simulink model "odev2"  (R2014a)
settings: Solver=ode45  StartTime=0.0  StopTime=10.0  RelTol=1e-3
undefined symbols (not defined in the file): gray, Rec, SDTV
libraries: visionconversions x18, visionsinks x14, visionsources x1
settings Model: Creator=bizimakin  LastModifiedBy=bizimakin
settings DebuggingCC: UnderspecifiedInitializationDetection=Classic  StateNameClashWarn=warning

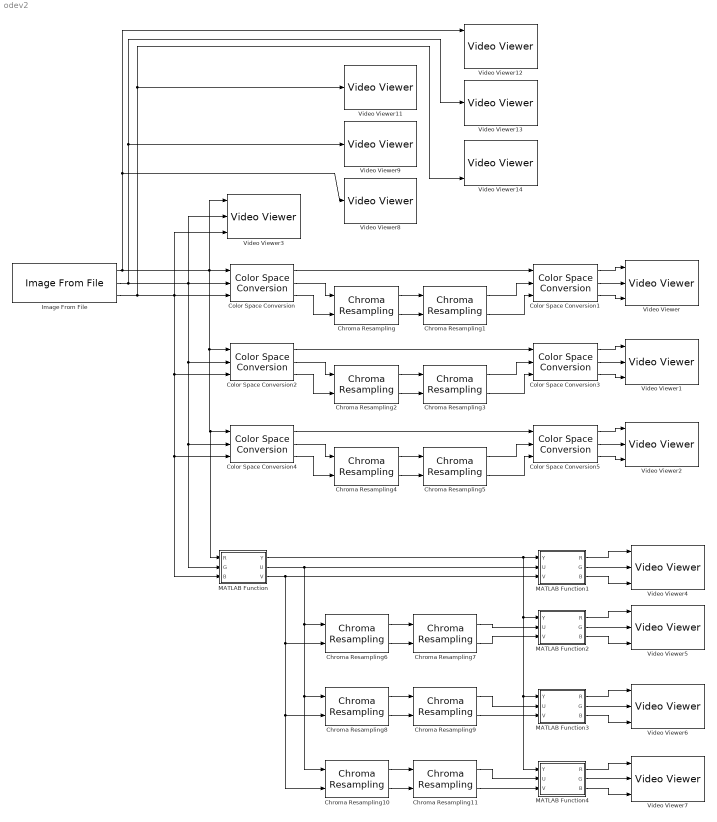
== system odev2 ==
  Chroma Resampling : visionconversions/Chroma Resampling  resampling=4:4:4 to 4:2:2  interpolation=pixel replication  antialiasing=Default  hcoeff=[0.2 0.6 0.2]  vcoeff=[0.5 0.5]  isInputTransposed=off
  Chroma Resampling1 : visionconversions/Chroma Resampling  resampling=4:2:2 to 4:4:4  interpolation=linear  antialiasing=Default  hcoeff=[0.2 0.6 0.2]  vcoeff=[0.5 0.5]  isInputTransposed=off
  Chroma Resampling10 : visionconversions/Chroma Resampling  resampling=4:4:4 to 4:2:0 (MPEG1)  interpolation=pixel replication  antialiasing=Default  hcoeff=[0.2 0.6 0.2]  vcoeff=[0.5 0.5]  isInputTransposed=off
  Chroma Resampling11 : visionconversions/Chroma Resampling  resampling=4:2:0 (MPEG1) to 4:4:4  interpolation=linear  antialiasing=Default  hcoeff=[0.2 0.6 0.2]  vcoeff=[0.5 0.5]  isInputTransposed=off
  Chroma Resampling2 : visionconversions/Chroma Resampling  resampling=4:4:4 to 4:1:1  interpolation=pixel replication  antialiasing=Default  hcoeff=[0.2 0.6 0.2]  vcoeff=[0.5 0.5]  isInputTransposed=off
  Chroma Resampling3 : visionconversions/Chroma Resampling  resampling=4:1:1 to 4:4:4  interpolation=linear  antialiasing=Default  hcoeff=[0.2 0.6 0.2]  vcoeff=[0.5 0.5]  isInputTransposed=off
  Chroma Resampling4 : visionconversions/Chroma Resampling  resampling=4:4:4 to 4:2:0 (MPEG1)  interpolation=pixel replication  antialiasing=Default  hcoeff=[0.2 0.6 0.2]  vcoeff=[0.5 0.5]  isInputTransposed=off
  Chroma Resampling5 : visionconversions/Chroma Resampling  resampling=4:2:0 (MPEG1) to 4:4:4  interpolation=linear  antialiasing=Default  hcoeff=[0.2 0.6 0.2]  vcoeff=[0.5 0.5]  isInputTransposed=off
  Chroma Resampling6 : visionconversions/Chroma Resampling  resampling=4:4:4 to 4:2:2  interpolation=pixel replication  antialiasing=Default  hcoeff=[0.2 0.6 0.2]  vcoeff=[0.5 0.5]  isInputTransposed=off
  Chroma Resampling7 : visionconversions/Chroma Resampling  resampling=4:2:2 to 4:4:4  interpolation=linear  antialiasing=Default  hcoeff=[0.2 0.6 0.2]  vcoeff=[0.5 0.5]  isInputTransposed=off
  Chroma Resampling8 : visionconversions/Chroma Resampling  resampling=4:4:4 to 4:1:1  interpolation=pixel replication  antialiasing=Default  hcoeff=[0.2 0.6 0.2]  vcoeff=[0.5 0.5]  isInputTransposed=off
  Chroma Resampling9 : visionconversions/Chroma Resampling  resampling=4:1:1 to 4:4:4  interpolation=linear  antialiasing=Default  hcoeff=[0.2 0.6 0.2]  vcoeff=[0.5 0.5]  isInputTransposed=off
  Color Space Conversion : visionconversions/Color Space  Conversion  conversion=Obsolete  conversionActive=R'G'B' to Y'CbCr  wp_str=D65  rec=Rec. 601 (SDTV)  sys=1125/60/2:1  imagePorts=Separate color signals
  Color Space Conversion1 : visionconversions/Color Space  Conversion  conversion=Obsolete  conversionActive=Y'CbCr to R'G'B'  wp_str=D65  rec=Rec. 601 (SDTV)  sys=1125/60/2:1  imagePorts=Separate color signals
  Color Space Conversion2 : visionconversions/Color Space  Conversion  conversion=Obsolete  conversionActive=R'G'B' to Y'CbCr  wp_str=D65  rec=Rec. 601 (SDTV)  sys=1125/60/2:1  imagePorts=Separate color signals
  Color Space Conversion3 : visionconversions/Color Space  Conversion  conversion=Obsolete  conversionActive=Y'CbCr to R'G'B'  wp_str=D65  rec=Rec. 601 (SDTV)  sys=1125/60/2:1  imagePorts=Separate color signals
  Color Space Conversion4 : visionconversions/Color Space  Conversion  conversion=Obsolete  conversionActive=R'G'B' to Y'CbCr  wp_str=D65  rec=Rec. 601 (SDTV)  sys=1125/60/2:1  imagePorts=Separate color signals
  Color Space Conversion5 : visionconversions/Color Space  Conversion  conversion=Obsolete  conversionActive=Y'CbCr to R'G'B'  wp_str=D65  rec=Rec. 601 (SDTV)  sys=1125/60/2:1  imagePorts=Separate color signals
  Image From File : visionsources/Image From File  Tag=vipblks_nd  FileName=C:\Users\bizimakin\Desktop\parrots.jpg  imagePorts=Separate color signals  Ts=inf  ImageDataType=double  Signed=on  WordLength=16  sdImageDataType=uint(8)  FractionLengthMode=User-defined  FractionLength=15  OutPortLabels=R|G|B
  MATLAB Function : MATLAB Function  TreatAsAtomicUnit=on
  MATLAB Function1 : MATLAB Function  TreatAsAtomicUnit=on
  MATLAB Function2 : MATLAB Function  TreatAsAtomicUnit=on
  MATLAB Function3 : MATLAB Function  TreatAsAtomicUnit=on
  MATLAB Function4 : MATLAB Function  TreatAsAtomicUnit=on
  Video Viewer{,12..14} (4 alike) : visionsinks/Video Viewer  inputType=Obsolete7b  imagePorts=Separate color signals  useColorMap=off  colormapValue=gray(256)  specRange=off  minInputVal=0  maxInputVal=255  FigPos=[193 561 410 300]  AxisZoom=on  trueSizedOnce=off  OpenAtMdlStart=on  DefaultConfigurationName=vipscopes.VideoViewerScopeCfg
  Video Viewer1 : visionsinks/Video Viewer  inputType=Obsolete7b  imagePorts=Separate color signals  useColorMap=off  colormapValue=gray(256)  specRange=off  minInputVal=0  maxInputVal=255  FigPos=[390 779 410 300]  AxisZoom=on  trueSizedOnce=off  OpenAtMdlStart=on  DefaultConfigurationName=vipscopes.VideoViewerScopeCfg
  Video Viewer11 : visionsinks/Video Viewer  inputType=Obsolete7b  imagePorts=One multidimensional signal  useColorMap=off  colormapValue=gray(256)  specRange=off  minInputVal=0  maxInputVal=255  FigPos=[787 651 410 300]  AxisZoom=on  trueSizedOnce=off  OpenAtMdlStart=on  DefaultConfigurationName=vipscopes.VideoViewerScopeCfg
  Video Viewer{2,4..7} (5 alike) : visionsinks/Video Viewer  inputType=Obsolete7b  imagePorts=Separate color signals  useColorMap=off  colormapValue=gray(256)  specRange=off  minInputVal=0  maxInputVal=255  FigPos=[663 467 410 300]  AxisZoom=on  trueSizedOnce=off  OpenAtMdlStart=on  DefaultConfigurationName=vipscopes.VideoViewerScopeCfg
  Video Viewer3 : visionsinks/Video Viewer  inputType=Obsolete7b  imagePorts=Separate color signals  useColorMap=off  colormapValue=gray(256)  specRange=off  minInputVal=0  maxInputVal=255  FigPos=[787 651 410 300]  AxisZoom=on  trueSizedOnce=off  OpenAtMdlStart=on  DefaultConfigurationName=vipscopes.VideoViewerScopeCfg
  Video Viewer8 : visionsinks/Video Viewer  inputType=Obsolete7b  imagePorts=One multidimensional signal  useColorMap=off  colormapValue=gray(256)  specRange=off  minInputVal=0  maxInputVal=255  FigPos=[308 631 410 300]  AxisZoom=on  trueSizedOnce=off  OpenAtMdlStart=on  DefaultConfigurationName=vipscopes.VideoViewerScopeCfg
  Video Viewer9 : visionsinks/Video Viewer  inputType=Obsolete7b  imagePorts=One multidimensional signal  useColorMap=off  colormapValue=gray(256)  specRange=off  minInputVal=0  maxInputVal=255  FigPos=[787 651 410 300]  AxisZoom=on  trueSizedOnce=off  OpenAtMdlStart=on  DefaultConfigurationName=vipscopes.VideoViewerScopeCfg
  wires:
  Color Space Conversion/1 -> Color Space Conversion1/1
  Color Space Conversion/2 -> Chroma Resampling/1
  Color Space Conversion/3 -> Chroma Resampling/2
  Color Space Conversion1/1 -> Video Viewer/1
  Chroma Resampling/1 -> Chroma Resampling1/1
  Chroma Resampling/2 -> Chroma Resampling1/2
  Color Space Conversion1/2 -> Video Viewer/2
  Color Space Conversion1/3 -> Video Viewer/3
  Chroma Resampling1/1 -> Color Space Conversion1/2
  Chroma Resampling1/2 -> Color Space Conversion1/3
  Image From File/2 -> Video Viewer9/1, Video Viewer13/2, Video Viewer3/2, MATLAB Function/2(G), Color Space Conversion4/2, Color Space Conversion2/2, Color Space Conversion/2
  Image From File/3 -> Video Viewer14/3, Video Viewer11/1, Video Viewer3/3, MATLAB Function/3(B), Color Space Conversion4/3, Color Space Conversion2/3, Color Space Conversion/3
  Image From File/1 -> Video Viewer12/1, Video Viewer8/1, Video Viewer3/1, MATLAB Function/1(R), Color Space Conversion4/1, Color Space Conversion2/1, Color Space Conversion/1
  Color Space Conversion2/1 -> Color Space Conversion3/1
  Color Space Conversion2/2 -> Chroma Resampling2/1
  Color Space Conversion2/3 -> Chroma Resampling2/2
  Color Space Conversion3/1 -> Video Viewer1/1
  Chroma Resampling2/1 -> Chroma Resampling3/1
  Chroma Resampling2/2 -> Chroma Resampling3/2
  Color Space Conversion3/2 -> Video Viewer1/2
  Color Space Conversion3/3 -> Video Viewer1/3
  Chroma Resampling3/1 -> Color Space Conversion3/2
  Chroma Resampling3/2 -> Color Space Conversion3/3
  Color Space Conversion4/1 -> Color Space Conversion5/1
  Color Space Conversion4/2 -> Chroma Resampling4/1
  Color Space Conversion4/3 -> Chroma Resampling4/2
  Color Space Conversion5/1 -> Video Viewer2/1
  Chroma Resampling4/1 -> Chroma Resampling5/1
  Chroma Resampling4/2 -> Chroma Resampling5/2
  Color Space Conversion5/2 -> Video Viewer2/2
  Color Space Conversion5/3 -> Video Viewer2/3
  Chroma Resampling5/1 -> Color Space Conversion5/2
  Chroma Resampling5/2 -> Color Space Conversion5/3
  MATLAB Function/1(Y) -> MATLAB Function4/1(Y), MATLAB Function3/1(Y), MATLAB Function2/1(Y), MATLAB Function1/1(Y)
  MATLAB Function/2(U) -> Chroma Resampling10/1, Chroma Resampling8/1, Chroma Resampling6/1, MATLAB Function1/2(U)
  MATLAB Function/3(V) -> Chroma Resampling10/2, Chroma Resampling8/2, Chroma Resampling6/2, MATLAB Function1/3(V)
  MATLAB Function1/1(R) -> Video Viewer4/1
  MATLAB Function1/2(G) -> Video Viewer4/2
  MATLAB Function1/3(B) -> Video Viewer4/3
  Chroma Resampling6/1 -> Chroma Resampling7/1
  Chroma Resampling6/2 -> Chroma Resampling7/2
  Chroma Resampling8/1 -> Chroma Resampling9/1
  Chroma Resampling8/2 -> Chroma Resampling9/2
  Chroma Resampling10/1 -> Chroma Resampling11/1
  Chroma Resampling10/2 -> Chroma Resampling11/2
  MATLAB Function2/1(R) -> Video Viewer5/1
  MATLAB Function2/2(G) -> Video Viewer5/2
  MATLAB Function2/3(B) -> Video Viewer5/3
  MATLAB Function3/1(R) -> Video Viewer6/1
  MATLAB Function3/2(G) -> Video Viewer6/2
  MATLAB Function3/3(B) -> Video Viewer6/3
  MATLAB Function4/1(R) -> Video Viewer7/1
  MATLAB Function4/2(G) -> Video Viewer7/2
  MATLAB Function4/3(B) -> Video Viewer7/3
  Chroma Resampling7/1 -> MATLAB Function2/2(U)
  Chroma Resampling7/2 -> MATLAB Function2/3(V)
  Chroma Resampling9/1 -> MATLAB Function3/2(U)
  Chroma Resampling9/2 -> MATLAB Function3/3(V)
  Chroma Resampling11/1 -> MATLAB Function4/2(U)
  Chroma Resampling11/2 -> MATLAB Function4/3(V)

== matlab function odev2/MATLAB Function1 ==
  data: R output; Y input; G output; B output; U input; V input
function [R,G,B] = fcn(Y,U,V)

   R = Y + 1.140*V;
   G = Y - 0.395*U - 0.581*V;
   B = Y + 2.032*U;

== matlab function odev2/MATLAB Function ==
  data: R input; Y output; G input; B input; U output; V output
function [Y,U,V] = fcn(R,G,B)

Y = 0.299*R + 0.587*G + 0.114*B;
U = 0.492*(B-Y);
V = 0.877*(R-Y);

== matlab function odev2/MATLAB Function2 ==
  data: R output; Y input; G output; B output; U input; V input
function [R,G,B] = fcn(Y,U,V)

   R = Y + 1.140*V;
   G = Y - 0.395*U - 0.581*V;
   B = Y + 2.032*U;

== matlab function odev2/MATLAB Function3 ==
  data: R output; Y input; G output; B output; U input; V input
function [R,G,B] = fcn(Y,U,V)

   R = Y + 1.140*V;
   G = Y - 0.395*U - 0.581*V;
   B = Y + 2.032*U;

== matlab function odev2/MATLAB Function4 ==
  data: R output; Y input; G output; B output; U input; V input
function [R,G,B] = fcn(Y,U,V)

   R = Y + 1.140*V;
   G = Y - 0.395*U - 0.581*V;
   B = Y + 2.032*U;
